simulink model "EV_Powertrain"  (R2023a)
settings: Solver=VariableStepAuto  StartTime=0.0  StopTime=10  RelTol=1e-3
values from neighbouring files (symbols this model uses):
  grade_deg = grades(k)    [Graph.m]
undefined symbols (not defined in the file or in its folder): canChannel
libraries: canmsglib x12, slpidlib x4, canlib x2
settings Model: Creator=MEHMET  LastModifiedBy=MEHMET
settings DataIOCC: SaveFormat=Array  ReturnWorkspaceOutputs=off

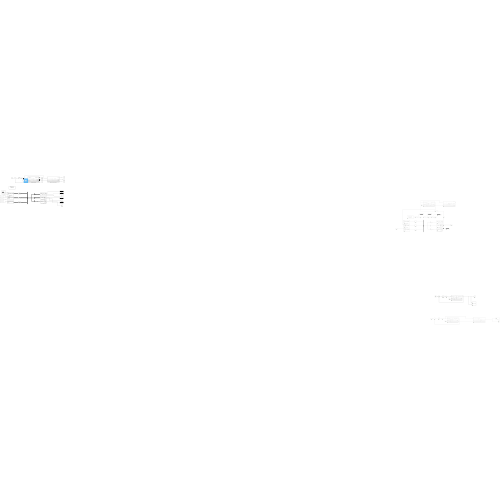
[thumbnail: Simulink's stored preview of the top-level diagram]
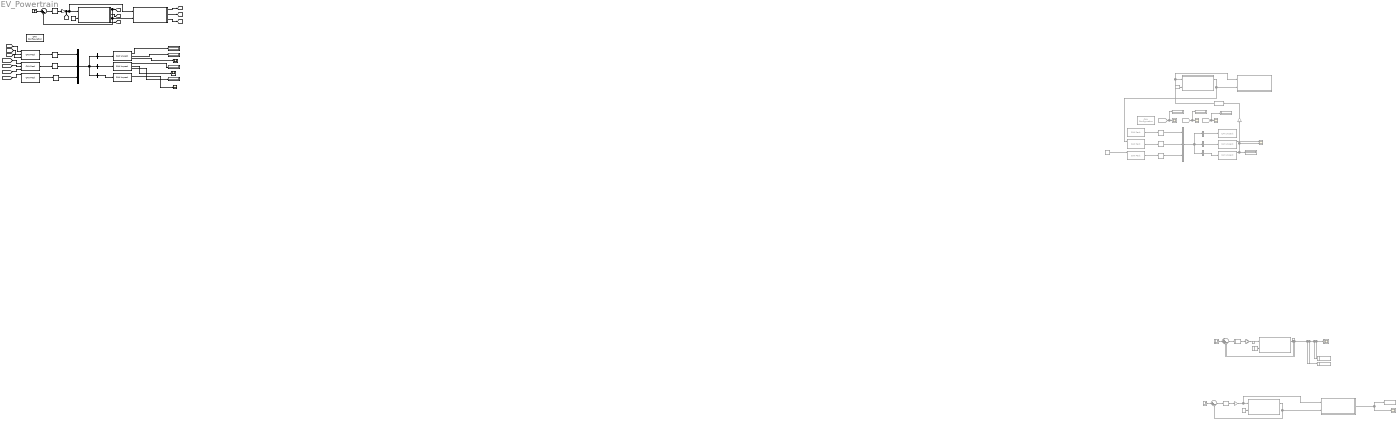
== system EV_Powertrain ==
  Acceleration : Scope
  Battery Energy Model Subsystem : Subsystem
  Battery Energy Modwl : Subsystem  Commented=on
  Battery Energy Modwl1 : Subsystem  Commented=on
  Battery Status : canmsglib/CAN Pack  Commented=on  MsgList=(none)  MsgName=Battery_Status  MsgIDType=Standard (11-bit identifier)  MsgIdentifier=100  MsgLength=8  Remote=off  ApplyMinMax=off  BusOutput=on  SignalInfo={ 'SOC', '0', '16', 'LE', 'unsigned', 'Standard', '0', '0.1', '0', '-Inf', 'Inf'; 'V_batt', '16', '16', 'LE', 'unsigned', 'Standard', '0', '0.1', '0', '-Inf', 'Inf'; 'I_batt', '32', '16', 'LE', 'unsigned', 'Standard', '0', '0.01', '0', '-Inf', 'Inf' }
      settings: LibrarySourceBlock=canlib/CAN Pack  DataFormat=manually specified signals
  Battery Status Unpack : canmsglib/CAN Unpack  Commented=on  MsgList=(none)  MsgName=Battery_Status  MsgIDType=Standard (11-bit identifier)  MsgIdentifier=100  MsgLength=8  SignalInfo={ 'SOC', '0', '16', 'LE', 'unsigned', 'Standard', '0', '0.1', '0', '-Inf', 'Inf'; 'V_batt', '16', '16', 'LE', 'unsigned', 'Standard', '0', '0.1', '0', '-Inf', 'Inf'; 'I_batt', '32', '16', 'LE', 'unsigned', 'Standard', '0', '0.01', '0', '-Inf', 'Inf' }  IDPort=off  TimestampPort=off  ErrorPort=off  RemotePort=off  LengthPort=off  StatusPort=off  ApplyMinMax=off
      settings: LibrarySourceBlock=canlib/CAN Unpack
  Battery Status Unpack1 : canmsglib/CAN Unpack  MsgList=(none)  MsgName=Battery_Status  MsgIDType=Standard (11-bit identifier)  MsgIdentifier=100  MsgLength=8  SignalInfo={ 'SOC', '0', '16', 'LE', 'unsigned', 'Standard', '0', '0.1', '0', '-Inf', 'Inf'; 'V_batt', '16', '16', 'LE', 'unsigned', 'Standard', '0', '0.1', '0', '-Inf', 'Inf'; 'I_batt', '32', '16', 'LE', 'unsigned', 'Standard', '0', '0.01', '0', '-Inf', 'Inf' }  IDPort=off  TimestampPort=off  ErrorPort=off  RemotePort=off  LengthPort=off  StatusPort=off  ApplyMinMax=off
      settings: LibrarySourceBlock=canlib/CAN Unpack
  Battery Status1 : canmsglib/CAN Pack  MsgList=(none)  MsgName=Battery_Status  MsgIDType=Standard (11-bit identifier)  MsgIdentifier=100  MsgLength=8  Remote=off  ApplyMinMax=off  BusOutput=on  SignalInfo={ 'SOC', '0', '16', 'LE', 'unsigned', 'Standard', '0', '0.1', '0', '-Inf', 'Inf'; 'V_batt', '16', '16', 'LE', 'unsigned', 'Standard', '0', '0.1', '0', '-Inf', 'Inf'; 'I_batt', '32', '16', 'LE', 'unsigned', 'Standard', '0', '0.01', '0', '-Inf', 'Inf' }
      settings: LibrarySourceBlock=canlib/CAN Pack  DataFormat=manually specified signals
  Bus Creator : BusCreator  Commented=on  Inputs=3
  Bus Creator1 : BusCreator  Inputs=3
  Bus Selector : BusSelector  Commented=on  OutputSignals=signal1
  Bus Selector1 : BusSelector  Commented=on  OutputSignals=signal2
  Bus Selector2 : BusSelector  Commented=on  OutputSignals=signal3
  Bus Selector3 : BusSelector  OutputSignals=signal1
  Bus Selector4 : BusSelector  OutputSignals=signal2
  Bus Selector5 : BusSelector  OutputSignals=signal3
  CAN Configuration : canlib/CAN Configuration  Commented=on  BlockHandle=253.0004  Device=MathWorks Virtual 1 (Channel 1)  DeviceMenu=MathWorks Virtual 1 (Channel 1)  ObjConstructor=canChannel('MathWorks', 'Virtual 1', 1)  BusSpeed=500000  EnableBitParameters=off  AckMode=Normal
  CAN Configuration1 : canlib/CAN Configuration  BlockHandle=254.0001  Device=MathWorks Virtual 1 (Channel 1)  DeviceMenu=MathWorks Virtual 1 (Channel 1)  ObjConstructor=canChannel('MathWorks', 'Virtual 1', 1)  BusSpeed=500000  EnableBitParameters=off  AckMode=Normal
  Constant{1..4} (4 alike) : Constant  Commented=on  Value=0
  Constant5 : Constant  Value=grade_deg
  Data Type Conversion : DataTypeConversion  Commented=on  OutDataTypeStr=double  SaturateOnIntegerOverflow=off  RndMeth=Floor
  Display{,1..2,8} (4 alike) : Display  Commented=on
  From3 : From  Commented=on  GotoTag=V_batt_tx
  From4 : From  Commented=on  GotoTag=I_batt_tx  TagVisibility=global
  From5 : From  Commented=on  GotoTag=SOC_tx  TagVisibility=global
  Gain : Gain  Commented=on  Gain=1/0.3
  Gain2 : Gain  Commented=on  Gain=50
  Gain4 : Gain  Commented=on  Gain=50
  Gain5 : Gain  Commented=on  Gain=50
  Gain6 : Gain  Gain=50
  Grade .Angle : Display
  I_batt : Scope
  PID Controller1 : slpidlib/PID Controller  Commented=on  Controller=PID  Form=Parallel  TimeDomain=Continuous-time  UseExternalTs=off  SampleTime=-1  IntegratorMethod=Forward Euler  FilterMethod=Forward Euler  ControllerParametersSource=internal  P=5  I=1  UseKiTs=off  D=2  N=100  UseFilter=on  TunerSelectOption=Transfer Function Based (PID Tuner App)  InitialConditionSource=internal  InitialConditionForIntegrator=0  InitialConditionForFilter=0  DifferentiatorICPrevScaledInput=0  ExternalReset=none  TrackingMode=off  Kt=1  LimitOutput=off  SatLimitsSource=internal  UpperSaturationLimit=inf  LowerSaturationLimit=-inf  LinearizeAsGain=on  AntiWindupMode=none  Kb=1  LimitIntegrator=off  UpperIntegratorSaturationLimit=inf  LowerIntegratorSaturationLimit=-inf  POutMin=[]  POutMax=[]  IOutMin=[]  IOutMax=[]  DOutMin=[]  DOutMax=[]  NOutMin=[]  NOutMax=[]  SumOutMin=[]  SumOutMax=[]  SaturationOutMin=[]  SaturationOutMax=[]  PParamMin=[]  PParamMax=[]  IParamMin=[]  IParamMax=[]  DParamMin=[]  DParamMax=[]  NParamMin=[]  NParamMax=[]  KbParamMin=[]  KbParamMax=[]  KtParamMin=[]  KtParamMax=[]  KbOutMin=[]  KbOutMax=[]  KtOutMin=[]  KtOutMax=[]  IntegratorOutMin=[]  IntegratorOutMax=[]  FilterOutMin=[]  FilterOutMax=[]  SumI1OutMin=[]  SumI1OutMax=[]  SumI2OutMin=[]  SumI2OutMax=[]  SumI3OutMin=[]  SumI3OutMax=[]  SumI4OutMin=[]  SumI4OutMax=[]  SumDOutMin=[]  SumDOutMax=[]  DifferentiatorOutMin=[]  DifferentiatorOutMax=[]  FilterDiffOutCoefMin=[]  FilterDiffOutCoefMax=[]  ReciprocalOutMin=[]  ReciprocalOutMax=[]  SumDenOutMin=[]  SumDenOutMax=[]  SumNumOutMin=[]  SumNumOutMax=[]  DivideOutMin=[]  DivideOutMax=[]  UdiffTsProdOutMin=[]  UdiffTsProdOutMax=[]  NTsProdOutMin=[]  NTsProdOutMax=[]  UintegralTsProdOutMin=[]  UintegralTsProdOutMax=[]  UngainTsProdOutMin=[]  UngainTsProdOutMax=[]  ClampingZeroOutDataTypeStr=Inherit: Inherit via back propagation  ClampingZeroOutMin=[]  ClampingZeroOutMax=[]  FilterDenConstantOutDataTypeStr=Inherit: Inherit via back propagation  FilterDenConstantOutMin=[]  FilterDenConstantOutMax=[]  PCopyOutDataTypeStr=Inherit: Inherit via back propagation  PCopyOutMin=[]  PCopyOutMax=[]  NCopyOutDataTypeStr=Inherit: Inherit via back propagation  NCopyOutMin=[]  NCopyOutMax=[]  IntegratorContinuousStateAttributes=''  IntegratorStateMustResolveToSignalObject=off  IntegratorRTWStateStorageClass=Auto  FilterContinuousStateAttributes=''  FilterStateMustResolveToSignalObject=off  FilterRTWStateStorageClass=Auto  ParallelPVariant=InternalParameters  IdealPVariant=Disabled  IVariant=InternalParameters  DVariant=InternalParameters  IntegratorVariant=Continuous  SatVariant=Disabled  AWVariant=Passthrough  PCopyVariant=Disabled  TRVariant=Disabled  FdbkBlocksVariant=Forward  IdealPFdbkVariant=Disabled  SatFdbkVariant=Disabled  DerivativeFilterVariant=ContFilter  NVariant=InternalParameters  NCopyVariant=Disabled  FilterICVariant=InternalICsFilter  IntegratorICVariant=InternalICs  ExternalResetVariant=Disabled  TRSumVariant=Passthrough  SumFdbkVariant=Disabled  SumVariant=Sum_PID  TsampFilterVariant=InternalTs  TsampNgainVariant=Passthrough  TsampIntegralVariant=Disabled_SignalSpec  ExternalSaturationOutDataTypeStr=Inherit: Same as second input
  PID Controller2 : slpidlib/PID Controller  Commented=on  Controller=PID  Form=Parallel  TimeDomain=Continuous-time  UseExternalTs=off  SampleTime=-1  IntegratorMethod=Forward Euler  FilterMethod=Forward Euler  ControllerParametersSource=internal  P=5.7  I=1  UseKiTs=off  D=1  N=100  UseFilter=on  TunerSelectOption=Transfer Function Based (PID Tuner App)  InitialConditionSource=internal  InitialConditionForIntegrator=0  InitialConditionForFilter=0  DifferentiatorICPrevScaledInput=0  ExternalReset=none  TrackingMode=off  Kt=1  LimitOutput=off  SatLimitsSource=internal  UpperSaturationLimit=inf  LowerSaturationLimit=-inf  LinearizeAsGain=on  AntiWindupMode=none  Kb=1  LimitIntegrator=off  UpperIntegratorSaturationLimit=inf  LowerIntegratorSaturationLimit=-inf  POutMin=[]  POutMax=[]  IOutMin=[]  IOutMax=[]  DOutMin=[]  DOutMax=[]  NOutMin=[]  NOutMax=[]  SumOutMin=[]  SumOutMax=[]  SaturationOutMin=[]  SaturationOutMax=[]  PParamMin=[]  PParamMax=[]  IParamMin=[]  IParamMax=[]  DParamMin=[]  DParamMax=[]  NParamMin=[]  NParamMax=[]  KbParamMin=[]  KbParamMax=[]  KtParamMin=[]  KtParamMax=[]  KbOutMin=[]  KbOutMax=[]  KtOutMin=[]  KtOutMax=[]  IntegratorOutMin=[]  IntegratorOutMax=[]  FilterOutMin=[]  FilterOutMax=[]  SumI1OutMin=[]  SumI1OutMax=[]  SumI2OutMin=[]  SumI2OutMax=[]  SumI3OutMin=[]  SumI3OutMax=[]  SumI4OutMin=[]  SumI4OutMax=[]  SumDOutMin=[]  SumDOutMax=[]  DifferentiatorOutMin=[]  DifferentiatorOutMax=[]  FilterDiffOutCoefMin=[]  FilterDiffOutCoefMax=[]  ReciprocalOutMin=[]  ReciprocalOutMax=[]  SumDenOutMin=[]  SumDenOutMax=[]  SumNumOutMin=[]  SumNumOutMax=[]  DivideOutMin=[]  DivideOutMax=[]  UdiffTsProdOutMin=[]  UdiffTsProdOutMax=[]  NTsProdOutMin=[]  NTsProdOutMax=[]  UintegralTsProdOutMin=[]  UintegralTsProdOutMax=[]  UngainTsProdOutMin=[]  UngainTsProdOutMax=[]  ClampingZeroOutDataTypeStr=Inherit: Inherit via back propagation  ClampingZeroOutMin=[]  ClampingZeroOutMax=[]  FilterDenConstantOutDataTypeStr=Inherit: Inherit via back propagation  FilterDenConstantOutMin=[]  FilterDenConstantOutMax=[]  PCopyOutDataTypeStr=Inherit: Inherit via back propagation  PCopyOutMin=[]  PCopyOutMax=[]  NCopyOutDataTypeStr=Inherit: Inherit via back propagation  NCopyOutMin=[]  NCopyOutMax=[]  IntegratorContinuousStateAttributes=''  IntegratorStateMustResolveToSignalObject=off  IntegratorRTWStateStorageClass=Auto  FilterContinuousStateAttributes=''  FilterStateMustResolveToSignalObject=off  FilterRTWStateStorageClass=Auto  ParallelPVariant=InternalParameters  IdealPVariant=Disabled  IVariant=InternalParameters  DVariant=InternalParameters  IntegratorVariant=Continuous  SatVariant=Disabled  AWVariant=Passthrough  PCopyVariant=Disabled  TRVariant=Disabled  FdbkBlocksVariant=Forward  IdealPFdbkVariant=Disabled  SatFdbkVariant=Disabled  DerivativeFilterVariant=ContFilter  NVariant=InternalParameters  NCopyVariant=Disabled  FilterICVariant=InternalICsFilter  IntegratorICVariant=InternalICs  ExternalResetVariant=Disabled  TRSumVariant=Passthrough  SumFdbkVariant=Disabled  SumVariant=Sum_PID  TsampFilterVariant=InternalTs  TsampNgainVariant=Passthrough  TsampIntegralVariant=Disabled_SignalSpec  ExternalSaturationOutDataTypeStr=Inherit: Same as second input
  PID Controller3 : slpidlib/PID Controller  Controller=PID  Form=Parallel  TimeDomain=Continuous-time  UseExternalTs=off  SampleTime=-1  IntegratorMethod=Forward Euler  FilterMethod=Forward Euler  ControllerParametersSource=internal  P=5.6  I=1  UseKiTs=off  D=0.3  N=100  UseFilter=on  TunerSelectOption=Transfer Function Based (PID Tuner App)  InitialConditionSource=internal  InitialConditionForIntegrator=0  InitialConditionForFilter=0  DifferentiatorICPrevScaledInput=0  ExternalReset=none  TrackingMode=off  Kt=1  LimitOutput=off  SatLimitsSource=internal  UpperSaturationLimit=inf  LowerSaturationLimit=-inf  LinearizeAsGain=on  AntiWindupMode=none  Kb=1  LimitIntegrator=off  UpperIntegratorSaturationLimit=inf  LowerIntegratorSaturationLimit=-inf  POutMin=[]  POutMax=[]  IOutMin=[]  IOutMax=[]  DOutMin=[]  DOutMax=[]  NOutMin=[]  NOutMax=[]  SumOutMin=[]  SumOutMax=[]  SaturationOutMin=[]  SaturationOutMax=[]  PParamMin=[]  PParamMax=[]  IParamMin=[]  IParamMax=[]  DParamMin=[]  DParamMax=[]  NParamMin=[]  NParamMax=[]  KbParamMin=[]  KbParamMax=[]  KtParamMin=[]  KtParamMax=[]  KbOutMin=[]  KbOutMax=[]  KtOutMin=[]  KtOutMax=[]  IntegratorOutMin=[]  IntegratorOutMax=[]  FilterOutMin=[]  FilterOutMax=[]  SumI1OutMin=[]  SumI1OutMax=[]  SumI2OutMin=[]  SumI2OutMax=[]  SumI3OutMin=[]  SumI3OutMax=[]  SumI4OutMin=[]  SumI4OutMax=[]  SumDOutMin=[]  SumDOutMax=[]  DifferentiatorOutMin=[]  DifferentiatorOutMax=[]  FilterDiffOutCoefMin=[]  FilterDiffOutCoefMax=[]  ReciprocalOutMin=[]  ReciprocalOutMax=[]  SumDenOutMin=[]  SumDenOutMax=[]  SumNumOutMin=[]  SumNumOutMax=[]  DivideOutMin=[]  DivideOutMax=[]  UdiffTsProdOutMin=[]  UdiffTsProdOutMax=[]  NTsProdOutMin=[]  NTsProdOutMax=[]  UintegralTsProdOutMin=[]  UintegralTsProdOutMax=[]  UngainTsProdOutMin=[]  UngainTsProdOutMax=[]  ClampingZeroOutDataTypeStr=Inherit: Inherit via back propagation  ClampingZeroOutMin=[]  ClampingZeroOutMax=[]  FilterDenConstantOutDataTypeStr=Inherit: Inherit via back propagation  FilterDenConstantOutMin=[]  FilterDenConstantOutMax=[]  PCopyOutDataTypeStr=Inherit: Inherit via back propagation  PCopyOutMin=[]  PCopyOutMax=[]  NCopyOutDataTypeStr=Inherit: Inherit via back propagation  NCopyOutMin=[]  NCopyOutMax=[]  IntegratorContinuousStateAttributes=''  IntegratorStateMustResolveToSignalObject=off  IntegratorRTWStateStorageClass=Auto  FilterContinuousStateAttributes=''  FilterStateMustResolveToSignalObject=off  FilterRTWStateStorageClass=Auto  ParallelPVariant=InternalParameters  IdealPVariant=Disabled  IVariant=InternalParameters  DVariant=InternalParameters  IntegratorVariant=Continuous  SatVariant=Disabled  AWVariant=Passthrough  PCopyVariant=Disabled  TRVariant=Disabled  FdbkBlocksVariant=Forward  IdealPFdbkVariant=Disabled  SatFdbkVariant=Disabled  DerivativeFilterVariant=ContFilter  NVariant=InternalParameters  NCopyVariant=Disabled  FilterICVariant=InternalICsFilter  IntegratorICVariant=InternalICs  ExternalResetVariant=Disabled  TRSumVariant=Passthrough  SumFdbkVariant=Disabled  SumVariant=Sum_PID  TsampFilterVariant=InternalTs  TsampNgainVariant=Passthrough  TsampIntegralVariant=Disabled_SignalSpec  ExternalSaturationOutDataTypeStr=Inherit: Same as second input
  PID Controller4 : slpidlib/PID Controller  Commented=on  Controller=PID  Form=Parallel  TimeDomain=Continuous-time  UseExternalTs=off  SampleTime=-1  IntegratorMethod=Forward Euler  FilterMethod=Forward Euler  ControllerParametersSource=internal  P=5.6  I=1  UseKiTs=off  D=0.3  N=100  UseFilter=on  TunerSelectOption=Transfer Function Based (PID Tuner App)  InitialConditionSource=internal  InitialConditionForIntegrator=0  InitialConditionForFilter=0  DifferentiatorICPrevScaledInput=0  ExternalReset=none  TrackingMode=off  Kt=1  LimitOutput=off  SatLimitsSource=internal  UpperSaturationLimit=inf  LowerSaturationLimit=-inf  LinearizeAsGain=on  AntiWindupMode=none  Kb=1  LimitIntegrator=off  UpperIntegratorSaturationLimit=inf  LowerIntegratorSaturationLimit=-inf  POutMin=[]  POutMax=[]  IOutMin=[]  IOutMax=[]  DOutMin=[]  DOutMax=[]  NOutMin=[]  NOutMax=[]  SumOutMin=[]  SumOutMax=[]  SaturationOutMin=[]  SaturationOutMax=[]  PParamMin=[]  PParamMax=[]  IParamMin=[]  IParamMax=[]  DParamMin=[]  DParamMax=[]  NParamMin=[]  NParamMax=[]  KbParamMin=[]  KbParamMax=[]  KtParamMin=[]  KtParamMax=[]  KbOutMin=[]  KbOutMax=[]  KtOutMin=[]  KtOutMax=[]  IntegratorOutMin=[]  IntegratorOutMax=[]  FilterOutMin=[]  FilterOutMax=[]  SumI1OutMin=[]  SumI1OutMax=[]  SumI2OutMin=[]  SumI2OutMax=[]  SumI3OutMin=[]  SumI3OutMax=[]  SumI4OutMin=[]  SumI4OutMax=[]  SumDOutMin=[]  SumDOutMax=[]  DifferentiatorOutMin=[]  DifferentiatorOutMax=[]  FilterDiffOutCoefMin=[]  FilterDiffOutCoefMax=[]  ReciprocalOutMin=[]  ReciprocalOutMax=[]  SumDenOutMin=[]  SumDenOutMax=[]  SumNumOutMin=[]  SumNumOutMax=[]  DivideOutMin=[]  DivideOutMax=[]  UdiffTsProdOutMin=[]  UdiffTsProdOutMax=[]  NTsProdOutMin=[]  NTsProdOutMax=[]  UintegralTsProdOutMin=[]  UintegralTsProdOutMax=[]  UngainTsProdOutMin=[]  UngainTsProdOutMax=[]  ClampingZeroOutDataTypeStr=Inherit: Inherit via back propagation  ClampingZeroOutMin=[]  ClampingZeroOutMax=[]  FilterDenConstantOutDataTypeStr=Inherit: Inherit via back propagation  FilterDenConstantOutMin=[]  FilterDenConstantOutMax=[]  PCopyOutDataTypeStr=Inherit: Inherit via back propagation  PCopyOutMin=[]  PCopyOutMax=[]  NCopyOutDataTypeStr=Inherit: Inherit via back propagation  NCopyOutMin=[]  NCopyOutMax=[]  IntegratorContinuousStateAttributes=''  IntegratorStateMustResolveToSignalObject=off  IntegratorRTWStateStorageClass=Auto  FilterContinuousStateAttributes=''  FilterStateMustResolveToSignalObject=off  FilterRTWStateStorageClass=Auto  ParallelPVariant=InternalParameters  IdealPVariant=Disabled  IVariant=InternalParameters  DVariant=InternalParameters  IntegratorVariant=Continuous  SatVariant=Disabled  AWVariant=Passthrough  PCopyVariant=Disabled  TRVariant=Disabled  FdbkBlocksVariant=Forward  IdealPFdbkVariant=Disabled  SatFdbkVariant=Disabled  DerivativeFilterVariant=ContFilter  NVariant=InternalParameters  NCopyVariant=Disabled  FilterICVariant=InternalICsFilter  IntegratorICVariant=InternalICs  ExternalResetVariant=Disabled  TRSumVariant=Passthrough  SumFdbkVariant=Disabled  SumVariant=Sum_PID  TsampFilterVariant=InternalTs  TsampNgainVariant=Passthrough  TsampIntegralVariant=Disabled_SignalSpec  ExternalSaturationOutDataTypeStr=Inherit: Same as second input
  SOC : Display
  SOC1 : Scope  Commented=on
  Scope{,1..4} (5 alike) : Scope  Commented=on
  Scope5 : Scope  Commented=on  NumInputPorts=2
  Step1 : Step  Commented=on  Time=0  After=20  SampleTime=0
  Step2 : Step  Commented=on  Time=0  After=20  SampleTime=0
  Step4 : Step  Commented=on  Time=0  After=20  SampleTime=0
  Step5 : Step  Time=0  After=20  SampleTime=0
  Sum1 : Sum  Commented=on  Inputs=|+-
  Sum2 : Sum  Commented=on  Inputs=|+-
  Sum4 : Sum  Commented=on  Inputs=|+-
  Sum5 : Sum  Inputs=|+-
  To Virtual Bus : SignalConversion  Commented=on  ConversionOutput=Nonvirtual bus  OverrideOpt=off
  To Virtual Bus1 : SignalConversion  Commented=on  ConversionOutput=Nonvirtual bus  OverrideOpt=off
  To Virtual Bus2 : SignalConversion  Commented=on  ConversionOutput=Nonvirtual bus  OverrideOpt=off
  To Virtual Bus3 : SignalConversion  ConversionOutput=Nonvirtual bus  OverrideOpt=off
  To Virtual Bus4 : SignalConversion  ConversionOutput=Nonvirtual bus  OverrideOpt=off
  To Virtual Bus5 : SignalConversion  ConversionOutput=Nonvirtual bus  OverrideOpt=off
  To Workspace : ToWorkspace  Commented=on  VariableName=speed_flat  SampleTime=-1
  To Workspace1 : ToWorkspace  Commented=on  VariableName=speed_grade  SampleTime=-1
  To Workspace2 : ToWorkspace  Commented=on  VariableName=speed_flat2  SampleTime=-1
  To Workspace3 : ToWorkspace  Commented=on  VariableName=speed_grade2  SampleTime=-1
  Torque Command : canmsglib/CAN Pack  Commented=on  MsgList=(none)  MsgName=Torque_Command  MsgIDType=Standard (11-bit identifier)  MsgIdentifier=300  MsgLength=8  Remote=off  ApplyMinMax=off  BusOutput=on  SignalInfo={ 'Torque_Req', '0', '16', 'LE', 'unsigned', 'Standard', '0', '1', '0', '-Inf', 'Inf'; 'Mode', '16', '8', 'LE', 'unsigned', 'Standard', '0', '1', '0', '-Inf', 'Inf'; 'Reserved', '24', '8', 'LE', 'unsigned', 'Standard', '0', '1', '0', '-Inf', 'Inf' }
      settings: LibrarySourceBlock=canlib/CAN Pack  DataFormat=manually specified signals
  Torque Command Unpack : canmsglib/CAN Unpack  Commented=on  MsgList=(none)  MsgName=Torque_Command  MsgIDType=Standard (11-bit identifier)  MsgIdentifier=300  MsgLength=8  SignalInfo={ 'Torque_Req', '0', '16', 'LE', 'unsigned', 'Standard', '0', '1', '0', '-Inf', 'Inf'; 'Mode', '16', '8', 'LE', 'unsigned', 'Standard', '0', '1', '0', '-Inf', 'Inf'; 'Reserved', '24', '8', 'LE', 'unsigned', 'Standard', '0', '1', '0', '-Inf', 'Inf' }  IDPort=off  TimestampPort=off  ErrorPort=off  RemotePort=off  LengthPort=off  StatusPort=off  ApplyMinMax=off
      settings: LibrarySourceBlock=canlib/CAN Unpack
  Torque Command Unpack1 : canmsglib/CAN Unpack  MsgList=(none)  MsgName=Torque_Command  MsgIDType=Standard (11-bit identifier)  MsgIdentifier=300  MsgLength=8  SignalInfo={ 'Torque_Req', '0', '16', 'LE', 'unsigned', 'Standard', '0', '0.1', '0', '-Inf', 'Inf'; 'Mode', '16', '8', 'LE', 'unsigned', 'Standard', '0', '1', '0', '-Inf', 'Inf'; 'Reserved', '24', '8', 'LE', 'unsigned', 'Standard', '0', '1', '0', '-Inf', 'Inf' }  IDPort=off  TimestampPort=off  ErrorPort=off  RemotePort=off  LengthPort=off  StatusPort=off  ApplyMinMax=off
      settings: LibrarySourceBlock=canlib/CAN Unpack
  Torque Command1 : canmsglib/CAN Pack  MsgList=(none)  MsgName=Torque_Command  MsgIDType=Standard (11-bit identifier)  MsgIdentifier=300  MsgLength=8  Remote=off  ApplyMinMax=off  BusOutput=on  SignalInfo={ 'Torque_Req', '0', '16', 'LE', 'unsigned', 'Standard', '0', '1', '0', '-Inf', 'Inf'; 'Mode', '16', '8', 'LE', 'unsigned', 'Standard', '0', '1', '0', '-Inf', 'Inf'; 'Reserved', '24', '8', 'LE', 'unsigned', 'Standard', '0', '1', '0', '-Inf', 'Inf' }
      settings: LibrarySourceBlock=canlib/CAN Pack  DataFormat=manually specified signals
  Torque Req : Scope
  Torque_Req_Command : Constant  Commented=on  Value=100
  V_batt : Display
  Vehicle Dynamics Subsystem : Subsystem
  Vehicle Speed : Display
  Vehicle Status : canmsglib/CAN Pack  Commented=on  MsgList=(none)  MsgName=Vehicle_State  MsgIDType=Standard (11-bit identifier)  MsgIdentifier=200  MsgLength=8  Remote=off  ApplyMinMax=off  BusOutput=on  SignalInfo={ 'Vehicle_Speed', '0', '16', 'LE', 'unsigned', 'Standard', '0', '0.1', '0', '-Inf', 'Inf'; 'Acceleration', '16', '16', 'LE', 'unsigned', 'Standard', '0', '0.01', '0', '-Inf', 'Inf'; 'Grade_Angle', '32', '16', 'LE', 'unsigned', 'Standard', '0', '0.1', '0', '-Inf', 'Inf' }
      settings: LibrarySourceBlock=canlib/CAN Pack  DataFormat=manually specified signals
  "Vehicle Status Unpack " : canmsglib/CAN Unpack  Commented=on  MsgList=(none)  MsgName=CAN Msg  MsgIDType=Standard (11-bit identifier)  MsgIdentifier=200  MsgLength=8  SignalInfo={ 'Vehicle_Speed', '0', '16', 'LE', 'unsigned', 'Standard', '0', '0.1', '0', '-Inf', 'Inf'; 'Acceleration', '16', '16', 'LE', 'unsigned', 'Standard', '0', '0.01', '0', '-Inf', 'Inf'; 'Grade_Angle', '32', '16', 'LE', 'unsigned', 'Standard', '0', '0.1', '0', '-Inf', 'Inf' }  IDPort=off  TimestampPort=off  ErrorPort=off  RemotePort=off  LengthPort=off  StatusPort=off  ApplyMinMax=off
      settings: LibrarySourceBlock=canlib/CAN Unpack
  Vehicle Status Unpack 1 : canmsglib/CAN Unpack  MsgList=(none)  MsgName=CAN Msg  MsgIDType=Standard (11-bit identifier)  MsgIdentifier=200  MsgLength=8  SignalInfo={ 'Vehicle_Speed', '0', '16', 'LE', 'unsigned', 'Standard', '0', '0.1', '0', '-Inf', 'Inf'; 'Acceleration', '16', '16', 'LE', 'unsigned', 'Standard', '0', '0.01', '0', '-Inf', 'Inf'; 'Grade_Angle', '32', '16', 'LE', 'unsigned', 'Standard', '0', '0.1', '0', '-Inf', 'Inf' }  IDPort=off  TimestampPort=off  ErrorPort=off  RemotePort=off  LengthPort=off  StatusPort=off  ApplyMinMax=off
      settings: LibrarySourceBlock=canlib/CAN Unpack
  Vehicle Status1 : canmsglib/CAN Pack  MsgList=(none)  MsgName=Vehicle_State  MsgIDType=Standard (11-bit identifier)  MsgIdentifier=200  MsgLength=8  Remote=off  ApplyMinMax=off  BusOutput=on  SignalInfo={ 'Vehicle_Speed', '0', '16', 'LE', 'unsigned', 'Standard', '0', '0.1', '0', '-Inf', 'Inf'; 'Acceleration', '16', '16', 'LE', 'unsigned', 'Standard', '0', '0.01', '0', '-Inf', 'Inf'; 'Grade_Angle', '32', '16', 'LE', 'unsigned', 'Standard', '0', '0.1', '0', '-Inf', 'Inf' }
      settings: LibrarySourceBlock=canlib/CAN Pack  DataFormat=manually specified signals
  soc_log1 : ToWorkspace  Commented=on  VariableName=soc_log  SampleTime=-1
  vehicle_dynamics1 : Subsystem  Commented=on
  vehicle_dynamics2 : Subsystem  Commented=on
  vehicle_dynamics3 : Subsystem  Commented=on
  vehicle_dynamics4 : Subsystem  Commented=on
  wires:
  Constant1/1 -> vehicle_dynamics1/2(grade_deg)
  PID Controller1/1 -> Gain4/1
  Gain4/1 -> Battery Energy Modwl/1(In1), vehicle_dynamics1/1(wheel_Torque_Nm)
  Step1/1 -> Sum1/1
  Sum1/1 -> PID Controller1/1
  vehicle_dynamics1/1(Vehicle_Speed_mps) -> Sum1/2, Battery Energy Modwl/2(In2)
  Battery Energy Modwl/1(Out1) -> soc_log1/1, SOC1/1
  vehicle_dynamics2/1(Vehicle_Speed_mps) -> Sum2/2, To Workspace1/1, To Workspace/1, Scope/1
  Gain5/1 -> vehicle_dynamics2/1(wheel_Torque_Nm)
  PID Controller2/1 -> Gain5/1
  Step2/1 -> Sum2/1
  Constant3/1 -> vehicle_dynamics2/2(grade_deg)
  Sum2/1 -> PID Controller2/1
  Constant2/1 -> vehicle_dynamics3/2(grade_deg)
  vehicle_dynamics3/1(Vehicle_Speed_mps) -> Vehicle Status/1, Battery Energy Modwl1/2(2)
  Sum4/1 -> PID Controller4/1
  Constant4/1 -> vehicle_dynamics4/2(grade_deg)
  Step4/1 -> Sum4/1
  PID Controller4/1 -> Gain2/1
  Gain2/1 -> vehicle_dynamics4/1(wheel_Torque_Nm)
  vehicle_dynamics4/1(Vehicle_Speed_mps) -> Scope1/1, To Workspace2/1, To Workspace3/1, Sum4/2
  Torque Command/1 -> To Virtual Bus2/1
  Vehicle Status/1 -> To Virtual Bus1/1
  Battery Status/1 -> To Virtual Bus/1
  From5/1 -> Display2/1, Scope4/1
  From3/1 -> Display/1, Scope2/1
  From4/1 -> Display1/1, Scope3/1
  To Virtual Bus1/1 -> Bus Creator/2
  Bus Creator/1 -> Bus Selector2/1, Bus Selector/1, Bus Selector1/1
  Bus Selector/1 -> Battery Status Unpack/1  "<signal1>"
  Bus Selector1/1 -> "Vehicle Status Unpack "/1  "<signal2>"
  Bus Selector2/1 -> Torque Command Unpack/1  "<signal3>"
  To Virtual Bus/1 -> Bus Creator/1
  To Virtual Bus2/1 -> Bus Creator/3
  Torque_Req_Command/1 -> Torque Command/1
  Torque Command Unpack/1 -> Display8/1, Scope5/2, Gain/1
  "Vehicle Status Unpack "/1 -> Scope5/1
  To Virtual Bus5/1 -> Bus Creator1/3
  To Virtual Bus3/1 -> Bus Creator1/1
  Bus Selector5/1 -> Torque Command Unpack1/1  "<signal3>"
  Vehicle Status1/1 -> To Virtual Bus4/1
  Torque Command1/1 -> To Virtual Bus5/1
  Gain6/1 -> [Torque_Req], Vehicle Dynamics Subsystem/1(whel_Torque_Nm), Battery Energy Model Subsystem/1(In1)
  To Virtual Bus4/1 -> Bus Creator1/2
  Bus Selector3/1 -> Battery Status Unpack1/1  "<signal1>"
  Bus Creator1/1 -> Bus Selector5/1, Bus Selector3/1, Bus Selector4/1
  Battery Status1/1 -> To Virtual Bus3/1
  Constant5/1 -> Vehicle Dynamics Subsystem/2(grade_deg)
  Sum5/1 -> PID Controller3/1
  Step5/1 -> Sum5/1
  Bus Selector4/1 -> Vehicle Status Unpack 1/1  "<signal2>"
  Vehicle Dynamics Subsystem/1(Vehicle_Speed_mps) -> [Vehicle_Speed], Battery Energy Model Subsystem/2(2), Sum5/2
  PID Controller3/1 -> Gain6/1
  Gain/1 -> Data Type Conversion/1
  Data Type Conversion/1 -> vehicle_dynamics3/1(Torque Command), Battery Energy Modwl1/1(In1)
  Battery Status Unpack1/1 -> SOC/1
  Battery Status Unpack1/2 -> V_batt/1
  Battery Status Unpack1/3 -> I_batt/1
  Vehicle Status Unpack 1/1 -> Vehicle Speed/1
  Vehicle Status Unpack 1/3 -> Grade .Angle/1
  Torque Command Unpack1/1 -> Torque Req/1
  Vehicle Status Unpack 1/2 -> Acceleration/1
  Battery Energy Model Subsystem/1(SOC_tx) -> [SOC_tx]
  [SOC_tx] -> Battery Status1/1
  Battery Energy Model Subsystem/2(V_batt_tx) -> [V_batt_tx]
  Battery Energy Model Subsystem/3(I_batt_tx) -> [I_batt_tx]
  [V_batt_tx] -> Battery Status1/2
  [I_batt_tx] -> Battery Status1/3
  [Vehicle_Speed] -> Vehicle Status1/1
  Vehicle Dynamics Subsystem/2(Acceleration) -> [Acceleration]
  [Acceleration] -> Vehicle Status1/2
  Vehicle Dynamics Subsystem/3(Grade Angle) -> [Grade_Angle]
  [Grade_Angle] -> Vehicle Status1/3
  [Torque_Req] -> Torque Command1/1

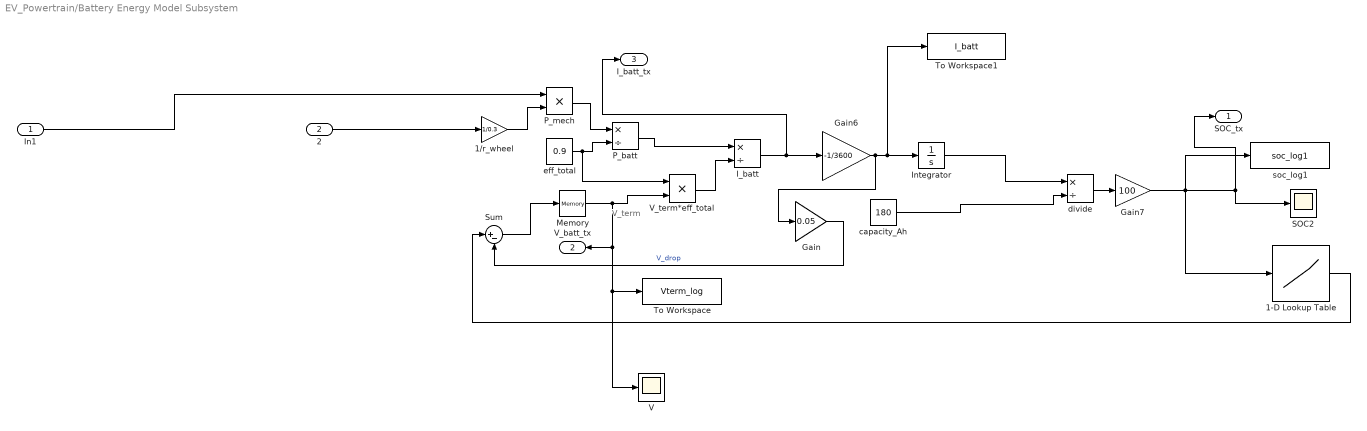
== system EV_Powertrain/Battery Energy Model Subsystem ==
  note: V_term
  In1 : Inport
  2 : Inport  Port=2
  1-D Lookup Table : Lookup_n-D  NumberOfTableDimensions=1  BreakpointsForDimension1=[10 20 40 60 80 100]  Table=[325 332 342 350 356 360]  InternalRulePriority=Speed  RndMeth=Simplest
  1/r_wheel : Gain  Gain=1/0.3
  Gain : Gain  Gain=0.05
  Gain6 : Gain  Gain=-1/3600
  Gain7 : Gain  Gain=100
  I_batt : Product  Inputs=*/  RndMeth=Zero  SaturateOnIntegerOverflow=on
  Integrator : Integrator  InitialCondition=180
  Memory : Memory  InitialCondition=0.01
  P_batt : Product  Inputs=*/
  P_mech : Product
  SOC2 : Scope
  Sum : Sum  Inputs=|+-
  To Workspace : ToWorkspace  VariableName=Vterm_log  SampleTime=-1
  To Workspace1 : ToWorkspace  VariableName=I_batt  SampleTime=-1
  V : Scope
  V_term*eff_total : Product
  capacity_Ah : Constant  Value=180
  divide : Product  Inputs=*/  RndMeth=Zero  SaturateOnIntegerOverflow=on
  eff_total : Constant  Value=0.9
  soc_log1 : ToWorkspace  VariableName=soc_log1  SampleTime=-1
  SOC_tx : Outport
  V_batt_tx : Outport  Port=2
  I_batt_tx : Outport  Port=3
  wires:
  Integrator/1 -> divide/1
  P_batt/1 -> I_batt/1
  2/1 -> 1/r_wheel/1
  In1/1 -> P_mech/1
  capacity_Ah/1 -> divide/2
  divide/1 -> Gain7/1
  1/r_wheel/1 -> P_mech/2
  P_mech/1 -> P_batt/1
  eff_total/1 -> V_term*eff_total/1, P_batt/2
  Gain7/1 -> soc_log1/1, 1-D Lookup Table/1, SOC_tx/1, SOC2/1
  1-D Lookup Table/1 -> Sum/1
  Memory/1 -> V_batt_tx/1, V/1, To Workspace/1, V_term*eff_total/2
  Sum/1 -> Memory/1
  I_batt/1 -> I_batt_tx/1, Gain6/1
  Gain6/1 -> To Workspace1/1, Integrator/1, Gain/1
  Gain/1 -> Sum/2  "V_drop"
  V_term*eff_total/1 -> I_batt/2

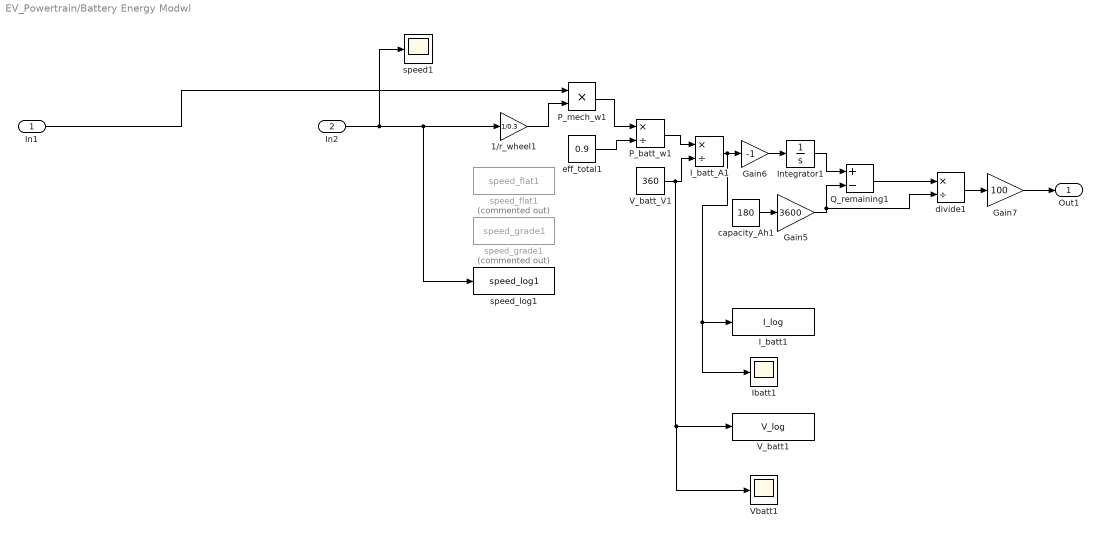
== system EV_Powertrain/Battery Energy Modwl ==
  In1 : Inport
  In2 : Inport  Port=2
  1/r_wheel1 : Gain  Gain=1/0.3
  Gain5 : Gain  Gain=3600
  Gain6 : Gain  Gain=-1
  Gain7 : Gain  Gain=100
  I_batt1 : ToWorkspace  VariableName=I_log  SampleTime=-1
  I_batt_A1 : Product  Inputs=*/  RndMeth=Zero  SaturateOnIntegerOverflow=on
  Ibatt1 : Scope
  Integrator1 : Integrator
  P_batt_w1 : Product  Inputs=*/
  P_mech_w1 : Product
  Q_remaining1 : Sum  Inputs=+-
  V_batt1 : ToWorkspace  VariableName=V_log  SampleTime=-1
  V_batt_V1 : Constant  Value=360
  Vbatt1 : Scope
  capacity_Ah1 : Constant  Value=180
  divide1 : Product  Inputs=*/  RndMeth=Zero  SaturateOnIntegerOverflow=on
  eff_total1 : Constant  Value=0.9
  speed1 : Scope
  speed_flat1 : ToWorkspace  Commented=on  VariableName=speed_flat1  SampleTime=-1
  speed_grade1 : ToWorkspace  Commented=on  VariableName=speed_grade1  SampleTime=-1
  speed_log1 : ToWorkspace  VariableName=speed_log1  SaveFormat=Timeseries  SampleTime=-1
  Out1 : Outport
  wires:
  V_batt_V1/1 -> Vbatt1/1, V_batt1/1, I_batt_A1/2
  Gain6/1 -> Integrator1/1
  Q_remaining1/1 -> divide1/1
  P_batt_w1/1 -> I_batt_A1/1
  In2/1 -> speed1/1, speed_log1/1, 1/r_wheel1/1
  capacity_Ah1/1 -> Gain5/1
  In1/1 -> P_mech_w1/1
  Gain5/1 -> Q_remaining1/2, divide1/2
  divide1/1 -> Gain7/1
  I_batt_A1/1 -> Ibatt1/1, I_batt1/1, Gain6/1
  1/r_wheel1/1 -> P_mech_w1/2
  Integrator1/1 -> Q_remaining1/1
  P_mech_w1/1 -> P_batt_w1/1
  eff_total1/1 -> P_batt_w1/2
  Gain7/1 -> Out1/1

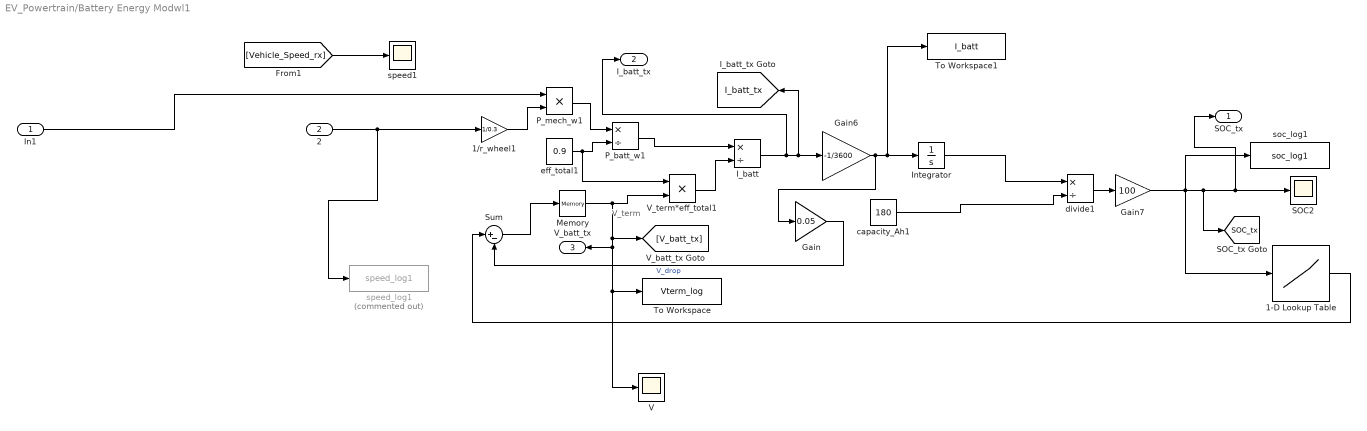
== system EV_Powertrain/Battery Energy Modwl1 ==
  note: V_term
  In1 : Inport
  2 : Inport  Port=2
  1-D Lookup Table : Lookup_n-D  NumberOfTableDimensions=1  BreakpointsForDimension1=[10 20 40 60 80 100]  Table=[325 332 342 350 356 360]  InternalRulePriority=Speed  RndMeth=Simplest
  1/r_wheel1 : Gain  Gain=1/0.3
  Gain : Gain  Gain=0.05
  Gain6 : Gain  Gain=-1/3600
  Gain7 : Gain  Gain=100
  I_batt : Product  Inputs=*/  RndMeth=Zero  SaturateOnIntegerOverflow=on
  Integrator : Integrator  InitialCondition=180
  Memory : Memory  InitialCondition=0.01
  P_batt_w1 : Product  Inputs=*/
  P_mech_w1 : Product
  SOC2 : Scope
  Sum : Sum  Inputs=|+-
  To Workspace : ToWorkspace  VariableName=Vterm_log  SampleTime=-1
  To Workspace1 : ToWorkspace  VariableName=I_batt  SampleTime=-1
  V : Scope
  V_term*eff_total1 : Product
  capacity_Ah1 : Constant  Value=180
  divide1 : Product  Inputs=*/  RndMeth=Zero  SaturateOnIntegerOverflow=on
  eff_total1 : Constant  Value=0.9
  soc_log1 : ToWorkspace  VariableName=soc_log1  SampleTime=-1
  speed1 : Scope
  speed_log1 : ToWorkspace  Commented=on  VariableName=speed_log1  SaveFormat=Timeseries  SampleTime=-1
  SOC_tx : Outport
  I_batt_tx : Outport  Port=2
  V_batt_tx : Outport  Port=3
  tag scope: I_batt_tx=global, SOC_tx=global
  wires:
  Integrator/1 -> divide1/1
  P_batt_w1/1 -> I_batt/1
  2/1 -> 1/r_wheel1/1, speed_log1/1
  In1/1 -> P_mech_w1/1
  capacity_Ah1/1 -> divide1/2
  divide1/1 -> Gain7/1
  1/r_wheel1/1 -> P_mech_w1/2
  P_mech_w1/1 -> P_batt_w1/1
  eff_total1/1 -> V_term*eff_total1/1, P_batt_w1/2
  Gain7/1 -> soc_log1/1, 1-D Lookup Table/1, SOC_tx/1, SOC2/1, [SOC_tx]
  1-D Lookup Table/1 -> Sum/1
  Memory/1 -> [V_batt_tx], V_batt_tx/1, V/1, To Workspace/1, V_term*eff_total1/2
  Sum/1 -> Memory/1
  I_batt/1 -> I_batt_tx/1, [I_batt_tx], Gain6/1
  Gain6/1 -> To Workspace1/1, Integrator/1, Gain/1
  Gain/1 -> Sum/2  "V_drop"
  V_term*eff_total1/1 -> I_batt/2
  [Vehicle_Speed_rx] -> speed1/1

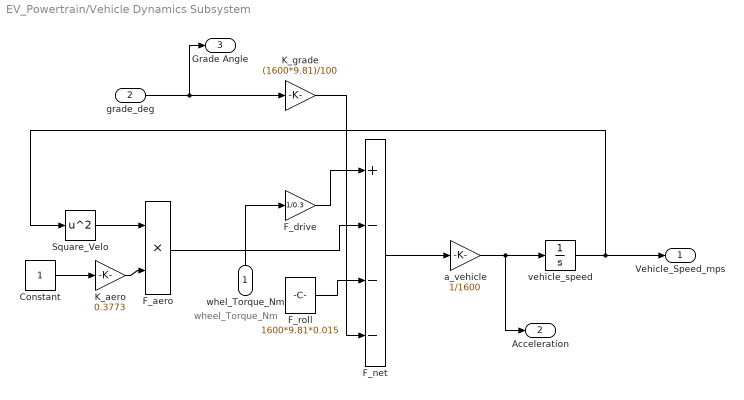
== system EV_Powertrain/Vehicle Dynamics Subsystem ==
  note: wheel_Torque_Nm
  whel_Torque_Nm : Inport
  grade_deg : Inport  Port=2
  Constant : Constant
  F_aero : Product
  F_drive : Gain  Gain=1/0.3
  F_net : Sum  Inputs=+---
  F_roll : Constant  Value=1600*9.81*0.015
  K_aero : Gain  Gain=0.3773
  K_grade : Gain  Gain=(1600*9.81)/100
  Square_Velo : Math  Operator=square
  a_vehicle : Gain  Gain=1/1600
  vehicle_speed : Integrator
  Vehicle_Speed_mps : Outport
  Acceleration : Outport  Port=2
  Grade Angle : Outport  Port=3
  wires:
  Square_Velo/1 -> F_aero/1
  grade_deg/1 -> Grade Angle/1, K_grade/1
  K_grade/1 -> F_net/4
  F_drive/1 -> F_net/1
  F_aero/1 -> F_net/2
  F_net/1 -> a_vehicle/1
  a_vehicle/1 -> Acceleration/1, vehicle_speed/1
  F_roll/1 -> F_net/3
  Constant/1 -> K_aero/1
  K_aero/1 -> F_aero/2
  vehicle_speed/1 -> Square_Velo/1, Vehicle_Speed_mps/1
  whel_Torque_Nm/1 -> F_drive/1

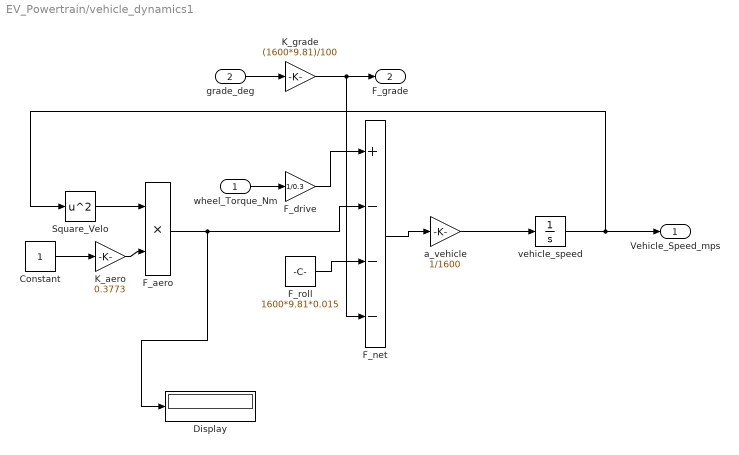
== system EV_Powertrain/vehicle_dynamics1 ==
  wheel_Torque_Nm : Inport
  grade_deg : Inport  Port=2
  Constant : Constant
  Display : Display
  F_aero : Product
  F_drive : Gain  Gain=1/0.3
  F_net : Sum  Inputs=+---
  F_roll : Constant  Value=1600*9.81*0.015
  K_aero : Gain  Gain=0.3773
  K_grade : Gain  Gain=(1600*9.81)/100
  Square_Velo : Math  Operator=square
  a_vehicle : Gain  Gain=1/1600
  vehicle_speed : Integrator
  Vehicle_Speed_mps : Outport
  F_grade : Outport  Port=2
  wires:
  Square_Velo/1 -> F_aero/1
  grade_deg/1 -> K_grade/1
  K_grade/1 -> F_net/4, F_grade/1
  F_drive/1 -> F_net/1
  F_aero/1 -> Display/1, F_net/2
  F_net/1 -> a_vehicle/1
  a_vehicle/1 -> vehicle_speed/1
  F_roll/1 -> F_net/3
  wheel_Torque_Nm/1 -> F_drive/1
  Constant/1 -> K_aero/1
  K_aero/1 -> F_aero/2
  vehicle_speed/1 -> Square_Velo/1, Vehicle_Speed_mps/1

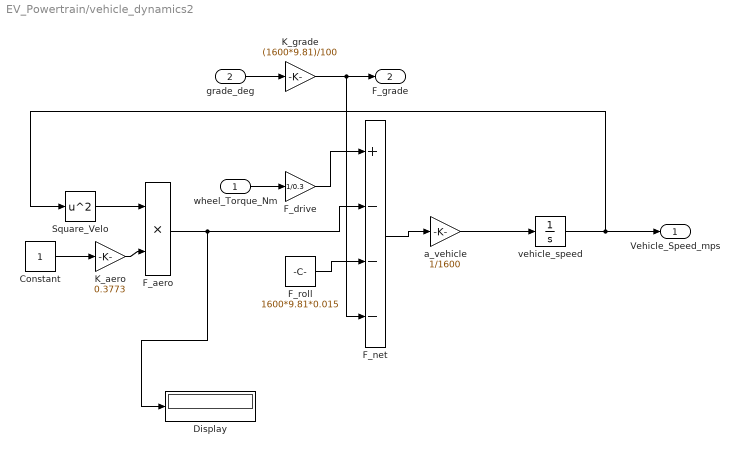
== system EV_Powertrain/vehicle_dynamics2 ==
  wheel_Torque_Nm : Inport
  grade_deg : Inport  Port=2
  Constant : Constant
  Display : Display
  F_aero : Product
  F_drive : Gain  Gain=1/0.3
  F_net : Sum  Inputs=+---
  F_roll : Constant  Value=1600*9.81*0.015
  K_aero : Gain  Gain=0.3773
  K_grade : Gain  Gain=(1600*9.81)/100
  Square_Velo : Math  Operator=square
  a_vehicle : Gain  Gain=1/1600
  vehicle_speed : Integrator
  Vehicle_Speed_mps : Outport
  F_grade : Outport  Port=2
  wires:
  Square_Velo/1 -> F_aero/1
  grade_deg/1 -> K_grade/1
  K_grade/1 -> F_net/4, F_grade/1
  F_drive/1 -> F_net/1
  F_aero/1 -> Display/1, F_net/2
  F_net/1 -> a_vehicle/1
  a_vehicle/1 -> vehicle_speed/1
  F_roll/1 -> F_net/3
  wheel_Torque_Nm/1 -> F_drive/1
  Constant/1 -> K_aero/1
  K_aero/1 -> F_aero/2
  vehicle_speed/1 -> Square_Velo/1, Vehicle_Speed_mps/1

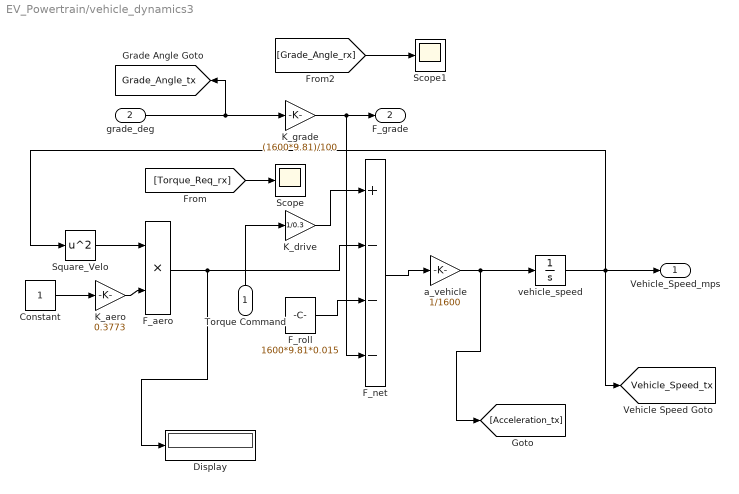
== system EV_Powertrain/vehicle_dynamics3 ==
  Torque Command : Inport
  grade_deg : Inport  Port=2
  Constant : Constant
  Display : Display
  F_aero : Product
  F_net : Sum  Inputs=+---
  F_roll : Constant  Value=1600*9.81*0.015
  K_aero : Gain  Gain=0.3773
  K_drive : Gain  Gain=1/0.3
  K_grade : Gain  Gain=(1600*9.81)/100
  Scope : Scope
  Scope1 : Scope
  Square_Velo : Math  Operator=square
  a_vehicle : Gain  Gain=1/1600
  vehicle_speed : Integrator
  Vehicle_Speed_mps : Outport
  F_grade : Outport  Port=2
  tag scope: Grade_Angle_tx=global, Vehicle_Speed_tx=global
  wires:
  Square_Velo/1 -> F_aero/1
  grade_deg/1 -> [Grade_Angle_tx], K_grade/1
  K_grade/1 -> F_net/4, F_grade/1
  K_drive/1 -> F_net/1
  F_aero/1 -> Display/1, F_net/2
  F_net/1 -> a_vehicle/1
  a_vehicle/1 -> [Acceleration_tx], vehicle_speed/1
  F_roll/1 -> F_net/3
  Constant/1 -> K_aero/1
  K_aero/1 -> F_aero/2
  vehicle_speed/1 -> [Vehicle_Speed_tx], Square_Velo/1, Vehicle_Speed_mps/1
  [Torque_Req_rx] -> Scope/1
  [Grade_Angle_rx] -> Scope1/1
  Torque Command/1 -> K_drive/1

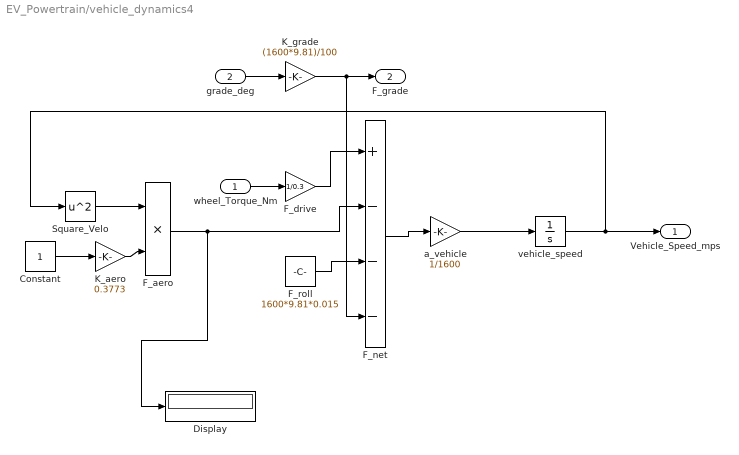
== system EV_Powertrain/vehicle_dynamics4 ==
  wheel_Torque_Nm : Inport
  grade_deg : Inport  Port=2
  Constant : Constant
  Display : Display
  F_aero : Product
  F_drive : Gain  Gain=1/0.3
  F_net : Sum  Inputs=+---
  F_roll : Constant  Value=1600*9.81*0.015
  K_aero : Gain  Gain=0.3773
  K_grade : Gain  Gain=(1600*9.81)/100
  Square_Velo : Math  Operator=square
  a_vehicle : Gain  Gain=1/1600
  vehicle_speed : Integrator
  Vehicle_Speed_mps : Outport
  F_grade : Outport  Port=2
  wires:
  vehicle_speed/1 -> Vehicle_Speed_mps/1, Square_Velo/1
  K_aero/1 -> F_aero/2
  Constant/1 -> K_aero/1
  wheel_Torque_Nm/1 -> F_drive/1
  F_roll/1 -> F_net/3
  a_vehicle/1 -> vehicle_speed/1
  F_net/1 -> a_vehicle/1
  F_aero/1 -> F_net/2, Display/1
  F_drive/1 -> F_net/1
  K_grade/1 -> F_grade/1, F_net/4
  grade_deg/1 -> K_grade/1
  Square_Velo/1 -> F_aero/1
